simulink subsystem "plant"  (R2025b)
settings: Solver=VariableStepAuto  StartTime=0.0  StopTime=10.0  RelTol=1e-3
undefined symbols (not defined in the file or in its folder): DiscIntNeverNeededParam, do_buoyancy_flag, do_drag_flag, do_force_flag, do_gravity_flag, do_thrusters_flag, do_time_flag, do_torque_flag, drag_wrench_lin, drag_wrench_quad, dt_data, dt_sim, FT_wrench, I, invI, invM, m, MT_wrench, R_cm2cv, rho, V_total, X0
settings Model: Creator=kjhaydon  LastModifiedBy=kjhaydon

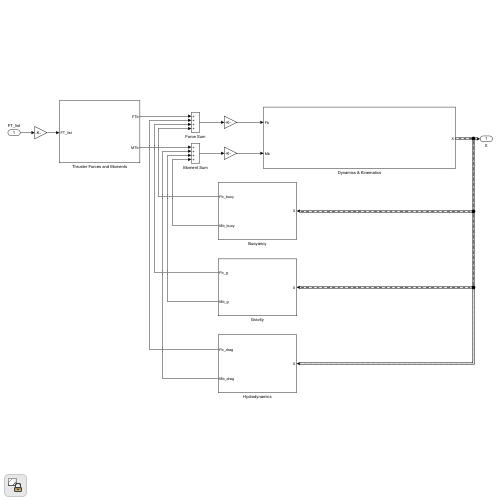
[thumbnail: Simulink's stored preview of the top-level diagram]
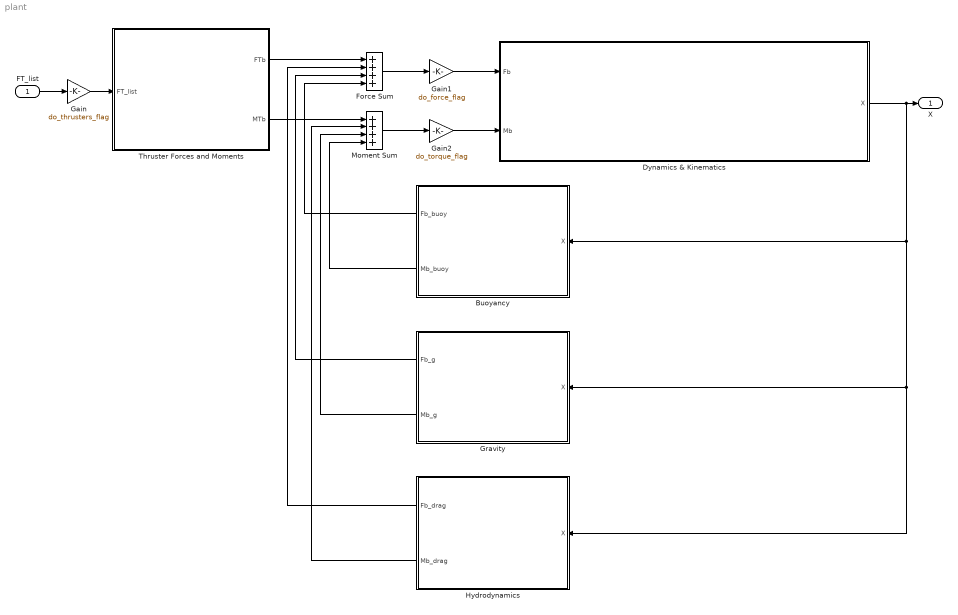
== system plant ==
  FT_list : Inport  SampleTime=dt_sim
  Buoyancy : Subsystem
  Dynamics & Kinematics : Subsystem
  Force Sum : Sum  Inputs=++++
  Gain : Gain  Gain=do_thrusters_flag
  Gain1 : Gain  Gain=do_force_flag
  Gain2 : Gain  Gain=do_torque_flag
  Gravity : Subsystem
  Hydrodynamics : Subsystem
  Moment Sum : Sum  Inputs=++++
  Thruster Forces and Moments : Subsystem
  X : Outport
  wires:
  Gravity/1(Fb_g) -> Force Sum/3
  Buoyancy/1(Fb_buoy) -> Force Sum/4
  Dynamics & Kinematics/1(X) -> X/1, Buoyancy/1(X), Gravity/1(X), Hydrodynamics/1(X)
  Buoyancy/2(Mb_buoy) -> Moment Sum/4
  Gravity/2(Mb_g) -> Moment Sum/3
  Gain/1 -> Thruster Forces and Moments/1(FT_list)
  Thruster Forces and Moments/2(MTb) -> Moment Sum/1
  FT_list/1 -> Gain/1
  Thruster Forces and Moments/1(FTb) -> Force Sum/1
  Force Sum/1 -> Gain1/1
  Gain1/1 -> Dynamics & Kinematics/1(Fb)
  Moment Sum/1 -> Gain2/1
  Hydrodynamics/2(Mb_drag) -> Moment Sum/2
  Hydrodynamics/1(Fb_drag) -> Force Sum/2
  Gain2/1 -> Dynamics & Kinematics/2(Mb)

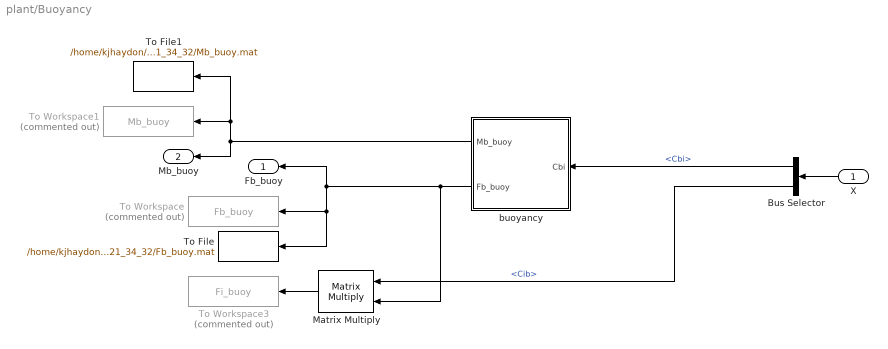
== system plant/Buoyancy ==
  X : Inport  OutDataTypeStr=Bus: X_bus
  Bus Selector : BusSelector  OutputSignals=Cbi,Cib
  Matrix Multiply : Product  Multiplication=Matrix(*)
  To File : ToFile  Filename=/home/kjhaydon/Github/Robosub/SimulinkPlant/data/2026_06_29_21_34_32/Fb_buoy.mat  MatrixName=Fb_buoy  SaveFormat=Timeseries  SampleTime=dt_data
  To File1 : ToFile  Filename=/home/kjhaydon/Github/Robosub/SimulinkPlant/data/2026_06_29_21_34_32/Mb_buoy.mat  MatrixName=Mb_buoy  SaveFormat=Timeseries  SampleTime=dt_data
  To Workspace : ToWorkspace  Commented=on  VariableName=Fb_buoy  SaveFormat=Timeseries  SampleTime=dt_data
  To Workspace1 : ToWorkspace  Commented=on  VariableName=Mb_buoy  SaveFormat=Timeseries  SampleTime=-1
  To Workspace3 : ToWorkspace  Commented=on  VariableName=Fi_buoy  SaveFormat=Timeseries  SampleTime=dt_data
  buoyancy : MATLAB Function  TreatAsAtomicUnit=on
  Fb_buoy : Outport
  Mb_buoy : Outport  Port=2
  wires:
  Bus Selector/1 -> buoyancy/1(Cbi)  "<Cbi>"
  X/1 -> Bus Selector/1
  Bus Selector/2 -> Matrix Multiply/1  "<Cib>"
  Matrix Multiply/1 -> To Workspace3/1
  buoyancy/1(Mb_buoy) -> To File1/1, To Workspace1/1, Mb_buoy/1
  buoyancy/2(Fb_buoy) -> Matrix Multiply/2, Fb_buoy/1, To File/1, To Workspace/1

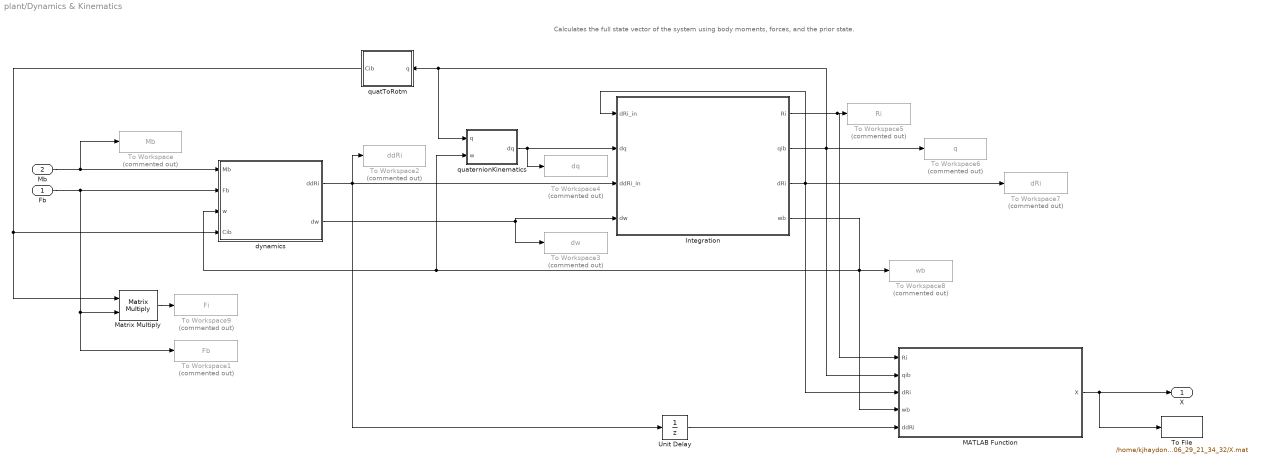
== system plant/Dynamics & Kinematics ==
  note: Calculates the full state vector of the system using body moments, forces, and the prior state.
  Fb : Inport
  Mb : Inport  Port=2
  Integration : Subsystem
  MATLAB Function : MATLAB Function  TreatAsAtomicUnit=on
  Matrix Multiply : Product  Multiplication=Matrix(*)
  To File : ToFile  Filename=/home/kjhaydon/Github/Robosub/SimulinkPlant/data/2026_06_29_21_34_32/X.mat  MatrixName=X  SaveFormat=Timeseries  SampleTime=dt_data
  To Workspace : ToWorkspace  Commented=on  VariableName=Mb  SaveFormat=Timeseries  SampleTime=dt_data
  To Workspace1 : ToWorkspace  Commented=on  VariableName=Fb  SaveFormat=Timeseries  SampleTime=dt_data
  To Workspace2 : ToWorkspace  Commented=on  VariableName=ddRi  SaveFormat=Timeseries  SampleTime=dt_data
  To Workspace3 : ToWorkspace  Commented=on  VariableName=dw  SaveFormat=Timeseries  SampleTime=dt_data
  To Workspace4 : ToWorkspace  Commented=on  VariableName=dq  SaveFormat=Timeseries  SampleTime=dt_data
  To Workspace5 : ToWorkspace  Commented=on  VariableName=Ri  SaveFormat=Timeseries  SampleTime=dt_data
  To Workspace6 : ToWorkspace  Commented=on  VariableName=q  SaveFormat=Timeseries  SampleTime=dt_data
  To Workspace7 : ToWorkspace  Commented=on  VariableName=dRi  SaveFormat=Timeseries  SampleTime=dt_data
  To Workspace8 : ToWorkspace  Commented=on  VariableName=wb  SaveFormat=Timeseries  SampleTime=dt_data
  To Workspace9 : ToWorkspace  Commented=on  VariableName=Fi  SaveFormat=Timeseries  SampleTime=dt_data
  Unit Delay : UnitDelay  InitialCondition=[0;0;0]  SampleTime=-1  HasFrameUpgradeWarning=on
  dynamics : MATLAB Function  TreatAsAtomicUnit=on
  quatToRotm : MATLAB Function  TreatAsAtomicUnit=on
  quaternionKinematics : MATLAB Function  TreatAsAtomicUnit=on
  X : Outport  OutDataTypeStr=Bus: X_bus
  wires:
  Unit Delay/1 -> MATLAB Function/5(ddRi)
  MATLAB Function/1(X) -> X/1, To File/1
  Matrix Multiply/1 -> To Workspace9/1
  quatToRotm/1(Cib) -> Matrix Multiply/1, dynamics/4(Cib)
  Fb/1 -> To Workspace1/1, Matrix Multiply/2, dynamics/2(Fb)
  dynamics/1(ddRi) -> Unit Delay/1, Integration/3(ddRi_in), To Workspace2/1
  dynamics/2(dw) -> To Workspace3/1, Integration/4(dw)
  Integration/3(dRi) -> To Workspace7/1, Integration/1(dRi_in), MATLAB Function/3(dRi)
  quaternionKinematics/1(dq) -> To Workspace4/1, Integration/2(dq)
  Integration/1(Ri) -> To Workspace5/1, MATLAB Function/1(Ri)
  Mb/1 -> dynamics/1(Mb), To Workspace/1
  Integration/2(qib) -> To Workspace6/1, quatToRotm/1(q), quaternionKinematics/1(q), MATLAB Function/2(qib)
  Integration/4(wb) -> MATLAB Function/4(wb), dynamics/3(w), quaternionKinematics/2(w), To Workspace8/1

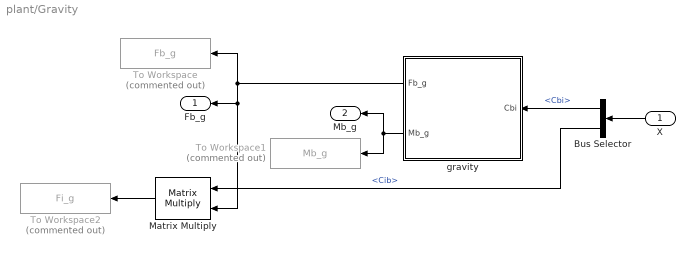
== system plant/Gravity ==
  X : Inport  OutDataTypeStr=Bus: X_bus
  Bus Selector : BusSelector  OutputSignals=Cbi,Cib
  Matrix Multiply : Product  Multiplication=Matrix(*)
  To Workspace : ToWorkspace  Commented=on  VariableName=Fb_g  SaveFormat=Timeseries  SampleTime=dt_data
  To Workspace1 : ToWorkspace  Commented=on  VariableName=Mb_g  SaveFormat=Timeseries  SampleTime=dt_data
  To Workspace2 : ToWorkspace  Commented=on  VariableName=Fi_g  SaveFormat=Timeseries  SampleTime=-1
  gravity : MATLAB Function  TreatAsAtomicUnit=on
  Fb_g : Outport
  Mb_g : Outport  Port=2
  wires:
  Bus Selector/2 -> Matrix Multiply/1  "<Cib>"
  Bus Selector/1 -> gravity/1(Cbi)  "<Cbi>"
  X/1 -> Bus Selector/1
  Matrix Multiply/1 -> To Workspace2/1
  gravity/2(Mb_g) -> Mb_g/1, To Workspace1/1
  gravity/1(Fb_g) -> To Workspace/1, Matrix Multiply/2, Fb_g/1

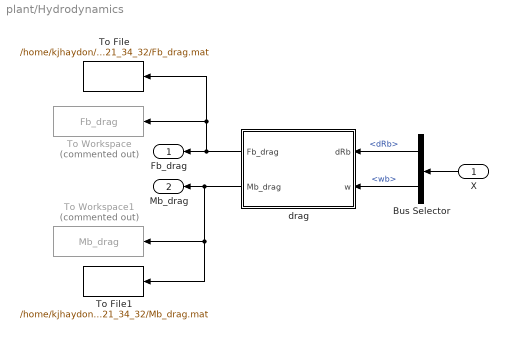
== system plant/Hydrodynamics ==
  X : Inport  OutDataTypeStr=Bus: X_bus
  Bus Selector : BusSelector  OutputSignals=dRb,wb
  To File : ToFile  Filename=/home/kjhaydon/Github/Robosub/SimulinkPlant/data/2026_06_29_21_34_32/Fb_drag.mat  MatrixName=Fb_drag  SaveFormat=Timeseries  SampleTime=dt_data
  To File1 : ToFile  Filename=/home/kjhaydon/Github/Robosub/SimulinkPlant/data/2026_06_29_21_34_32/Mb_drag.mat  MatrixName=Mb_drag  SaveFormat=Timeseries  SampleTime=dt_data
  To Workspace : ToWorkspace  Commented=on  VariableName=Fb_drag  SaveFormat=Timeseries  SampleTime=dt_data
  To Workspace1 : ToWorkspace  Commented=on  VariableName=Mb_drag  SaveFormat=Timeseries  SampleTime=dt_data
  drag : MATLAB Function  TreatAsAtomicUnit=on
  Fb_drag : Outport
  Mb_drag : Outport  Port=2
  wires:
  Bus Selector/2 -> drag/2(w)  "<wb>"
  Bus Selector/1 -> drag/1(dRb)  "<dRb>"
  X/1 -> Bus Selector/1
  drag/1(Fb_drag) -> Fb_drag/1, To File/1, To Workspace/1
  drag/2(Mb_drag) -> Mb_drag/1, To File1/1, To Workspace1/1

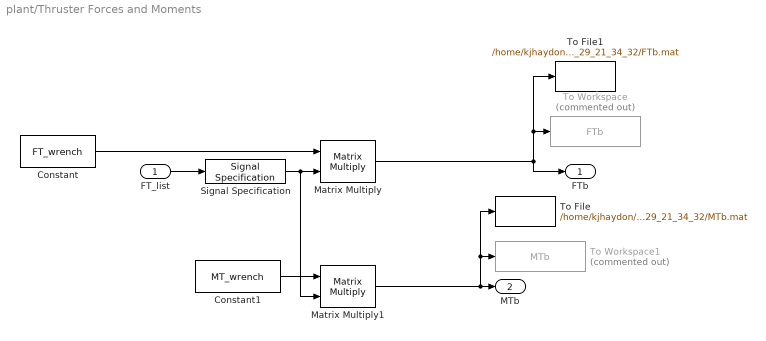
== system plant/Thruster Forces and Moments ==
  FT_list : Inport
  Constant : Constant  Value=FT_wrench
  Constant1 : Constant  Value=MT_wrench
  Matrix Multiply : Product  Multiplication=Matrix(*)
  Matrix Multiply1 : Product  Multiplication=Matrix(*)
  Signal Specification : SignalSpecification  Dimensions=[8 1]
  To File : ToFile  Filename=/home/kjhaydon/Github/Robosub/SimulinkPlant/data/2026_06_29_21_34_32/MTb.mat  MatrixName=MTb  SaveFormat=Timeseries  SampleTime=dt_data
  To File1 : ToFile  Filename=/home/kjhaydon/Github/Robosub/SimulinkPlant/data/2026_06_29_21_34_32/FTb.mat  MatrixName=FTb  SaveFormat=Timeseries  SampleTime=dt_data
  To Workspace : ToWorkspace  Commented=on  VariableName=FTb  SaveFormat=Timeseries  SampleTime=dt_data
  To Workspace1 : ToWorkspace  Commented=on  VariableName=MTb  SaveFormat=Timeseries  SampleTime=dt_data
  FTb : Outport
  MTb : Outport  Port=2
  wires:
  Matrix Multiply1/1 -> MTb/1, To Workspace1/1, To File/1
  Matrix Multiply/1 -> To File1/1, To Workspace/1, FTb/1
  Signal Specification/1 -> Matrix Multiply1/2, Matrix Multiply/2
  FT_list/1 -> Signal Specification/1
  Constant1/1 -> Matrix Multiply1/1
  Constant/1 -> Matrix Multiply/1

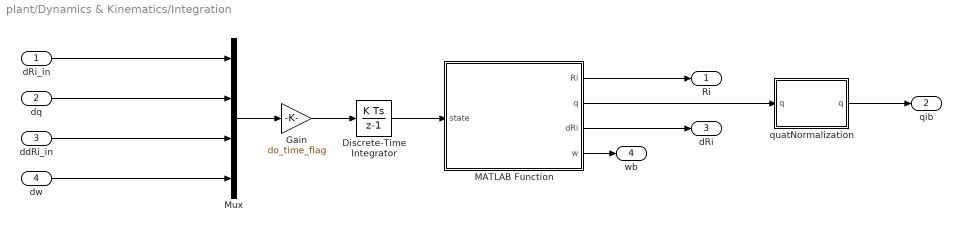
== system plant/Dynamics & Kinematics/Integration ==
  dRi_in : Inport
  dq : Inport  Port=2
  ddRi_in : Inport  Port=3
  dw : Inport  Port=4
  Discrete-Time Integrator : DiscreteIntegrator  InitialCondition=X0  SampleTime=-1  ICPrevOutput=DiscIntNeverNeededParam  ICPrevScaledInput=DiscIntNeverNeededParam
  Gain : Gain  Gain=do_time_flag
  MATLAB Function : MATLAB Function  TreatAsAtomicUnit=on
  Mux : Mux
  quatNormalization : MATLAB Function  TreatAsAtomicUnit=on
  Ri : Outport
  qib : Outport  Port=2
  dRi : Outport  Port=3
  wb : Outport  Port=4
  wires:
  Discrete-Time Integrator/1 -> MATLAB Function/1(state)
  Gain/1 -> Discrete-Time Integrator/1
  Mux/1 -> Gain/1
  MATLAB Function/2(q) -> quatNormalization/1("q ")
  quatNormalization/1(q) -> qib/1
  MATLAB Function/4(w) -> wb/1
  MATLAB Function/3(dRi) -> dRi/1
  MATLAB Function/1(Ri) -> Ri/1
  dRi_in/1 -> Mux/1
  dq/1 -> Mux/2
  dw/1 -> Mux/4
  ddRi_in/1 -> Mux/3

== matlab function plant/Hydrodynamics/drag ==
  data: dRb input; Fb_drag output; w input; Mb_drag output; drag_wrench_lin parameter; do_drag_flag parameter; drag_wrench_quad parameter
function [Fb_drag,Mb_drag] = fcn(dRb, w, drag_wrench_lin, do_drag_flag, drag_wrench_quad)

[Fb_drag, Mb_drag] = drag(dRb, w, drag_wrench_lin, drag_wrench_quad, do_drag_flag);

== matlab function plant/Dynamics & Kinematics/Integration/quatNormalization ==
  data: q input; q output
function q = fcn(q)

q = quatNormalization(q);

== matlab function plant/Dynamics & Kinematics/Integration/MATLAB Function ==
  data: Ri output; q output; dRi output; w output; state input
function [Ri,q,dRi,w] = fcn(state)
Ri = state(1:3);
q = state(4:7);
dRi = state(8:10);
w = state(11:13);
end

== matlab function plant/Buoyancy/buoyancy ==
  data: Mb_buoy output; Fb_buoy output; rho parameter; V_total parameter; R_cm2cv parameter; Cbi input; do_buoyancy_flag parameter
function [Mb_buoy,Fb_buoy] = fcn(rho, V_total, R_cm2cv,   Cbi, do_buoyancy_flag)

[Fb_buoy, Mb_buoy] =  buoyancy(Cbi, rho, V_total, R_cm2cv, do_buoyancy_flag);

== matlab function plant/Dynamics & Kinematics/MATLAB Function ==
  data: X output Bus: X_bus; Ri input; qib input; dRi input; wb input; ddRi input
function X = fcn(Ri, qib, dRi, wb, ddRi)

X = packStateIntoBus(Ri, qib, dRi, wb, ddRi);

== matlab function plant/Dynamics & Kinematics/dynamics ==
  data: Mb input; ddRi output; Fb input; w input; Cib input; dw output; I parameter; invM parameter; invI parameter
function [ddRi, dw] = fcn(Mb, Fb, w, Cib, I, invM, invI)

[ddRi,dw] = dynamics(Mb,Fb,w,Cib,I,invM,invI);

== matlab function plant/Dynamics & Kinematics/quatToRotm ==
  data: q input; Cib output
function Cib = fcn(q)

Cib = quatToRotm(q);

== matlab function plant/Dynamics & Kinematics/quaternionKinematics ==
  data: q input; dq output; w input
function dq = fcn(q,w)

dq = quaternionKinematics(q,w);

== matlab function plant/Gravity/gravity ==
  data: Cbi input; Fb_g output; Mb_g output; m parameter; do_gravity_flag parameter
function [Fb_g, Mb_g] = fcn(Cbi, m, do_gravity_flag)

[Fb_g, Mb_g] = gravity(Cbi, m, do_gravity_flag);
